simulink model "lidarUseModel"  (R2016a)
settings: Solver=ode15s  StartTime=0.0  StopTime=0.1  RelTol=1e-3
settings Model: Creator=mnorrito  LastModifiedBy=mnorrito
settings DataIOCC: SaveOutput=off  SaveTime=off

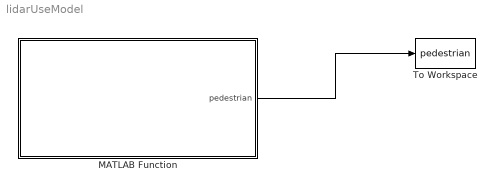
== system lidarUseModel ==
  MATLAB Function : MATLAB Function  TreatAsAtomicUnit=on
  To Workspace : ToWorkspace  VariableName=pedestrian  SaveFormat=Timeseries  SampleTime=-1
  wires:
  MATLAB Function/1(pedestrian) -> To Workspace/1

== matlab function lidarUseModel/MATLAB Function ==
  data: pedestrian output
function pedestrian = lidarUseModel()
coder.extrinsic('evalin')

  lidMatrix = cell(1,120);
  for i=1:120
      lidMatrix{i} = 0;
  end
  lidMatrix = evalin('base','lidMatrix');
  
  len = length(lidMatrix);
 
  pedestrian = 0;
  for coordIndex = 1:len/4
    beamLength = sqrt(lidMatrix{4*(coordIndex-1)+1}^2 + lidMatrix{4*(coordIndex-1)+2}^2);
    if(beamLength<20)
      if((4*(coordIndex)+1) <= len)
        beamLength = sqrt(lidMatrix{4*(coordIndex)+1}^2 + lidMatrix{4*(coordIndex)+2}^2);
      end
      if(beamLength<19)
        pedestrian = 1;
        break
      end
    end
  end
  
  
  
end
